simulink model "simpleTest"  (R2014a)
settings: Solver=ode45  StartTime=0.0  StopTime=10.0  RelTol=1e-3
values from neighbouring files (symbols this model uses):
  A = [0 3 4 ... (first row only)    [BJDF.m]
  B = [1;1;1]    [BJDF.m]
  C = [0 1 0;0 0 1]    [BJDF.m]
  D = [9 18;7 6;2 9]    [BJDF.m]
  f = 10    [BJDF.m]
  f1 = [-3 1 0]'    [BJDF.m]
  f2 = [1 -1/2 1/2]'    [BJDF.m]
  k = place(A,B,[-10,-11,-12])    [BJDF.m]
  pCV = CV*inv(CV'*CV)*CV'    [BJDF.m]
undefined symbols (not defined in the file or in its folder): magnitude
settings Model: Creator=sqn4594  LastModifiedBy=sqn4594

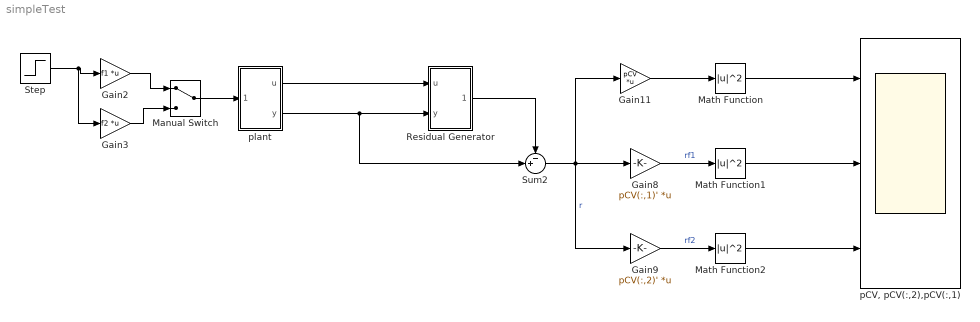
== system simpleTest ==
  Gain11 : Gain  Gain=pCV  Multiplication=Matrix(K*u)
  Gain2 : Gain  Gain=f1  Multiplication=Matrix(K*u)
  Gain3 : Gain  Gain=f2  Multiplication=Matrix(K*u)
  Gain8 : Gain  Gain=pCV(:,1)'  Multiplication=Matrix(K*u)
  Gain9 : Gain  Gain=pCV(:,2)'  Multiplication=Matrix(K*u)
  Manual Switch : ManualSwitch
  Math Function : Math  Operator=magnitude^2  SaturateOnIntegerOverflow=on
  Math Function1 : Math  Operator=magnitude^2  SaturateOnIntegerOverflow=on
  Math Function2 : Math  Operator=magnitude^2  SaturateOnIntegerOverflow=on
  Residual Generator : Subsystem
  Step : Step  Time=2  After=f  SampleTime=0
  Sum2 : Sum  Inputs=-+|
  "pCV, pCV(:,2),pCV(:,1)" : Scope  NumInputPorts=3
      settings: YMin=-5~-5~-5  YMax=5~5~5
  plant : Subsystem
  wires:
  Gain2/1 -> Manual Switch/1
  Gain3/1 -> Manual Switch/2
  Step/1 -> Gain3/1, Gain2/1
  Sum2/1 -> Gain11/1, Gain9/1, Gain8/1  "r"
  Gain8/1 -> Math Function1/1  "rf1"
  Gain9/1 -> Math Function2/1  "rf2"
  Math Function/1 -> "pCV, pCV(:,2),pCV(:,1)"/1
  Math Function1/1 -> "pCV, pCV(:,2),pCV(:,1)"/2
  Math Function2/1 -> "pCV, pCV(:,2),pCV(:,1)"/3
  Gain11/1 -> Math Function/1
  plant/2(y) -> Sum2/2, Residual Generator/2(y)
  Manual Switch/1 -> plant/1(f1/f2)
  plant/1(u) -> Residual Generator/1(u)
  Residual Generator/1(yHat) -> Sum2/1

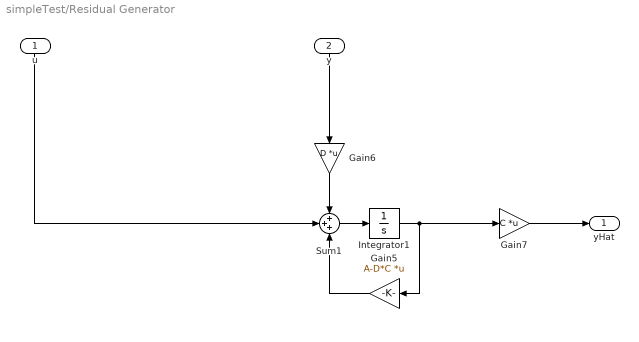
== system simpleTest/Residual Generator ==
  u : Inport
  y : Inport  Port=2
  Gain5 : Gain  Gain=A-D*C  Multiplication=Matrix(K*u)
  Gain6 : Gain  Gain=D  Multiplication=Matrix(K*u)
  Gain7 : Gain  Gain=C  Multiplication=Matrix(K*u)
  Integrator1 : Integrator
  Sum1 : Sum  Inputs=+++
  yHat : Outport
  wires:
  Gain6/1 -> Sum1/1
  Sum1/1 -> Integrator1/1
  Integrator1/1 -> Gain7/1, Gain5/1
  Gain5/1 -> Sum1/3
  Gain7/1 -> yHat/1
  u/1 -> Sum1/2
  y/1 -> Gain6/1

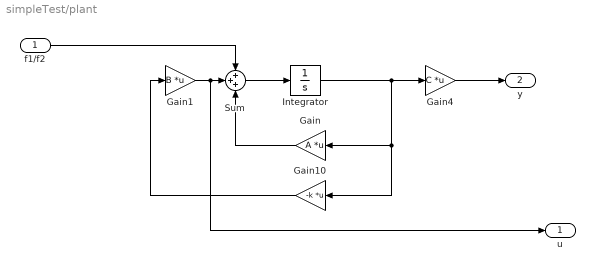
== system simpleTest/plant ==
  f1/f2 : Inport
  Gain : Gain  Gain=A  Multiplication=Matrix(K*u)
  Gain1 : Gain  Gain=B  Multiplication=Matrix(K*u)
  Gain10 : Gain  Gain=-k  Multiplication=Matrix(K*u)
  Gain4 : Gain  Gain=C  Multiplication=Matrix(K*u)
  Integrator : Integrator
  Sum : Sum  Inputs=+++
  u : Outport
  y : Outport  Port=2
  wires:
  Sum/1 -> Integrator/1
  Gain/1 -> Sum/3
  Gain1/1 -> u/1, Sum/2
  f1/f2/1 -> Sum/1
  Gain4/1 -> y/1
  Integrator/1 -> Gain4/1, Gain10/1, Gain/1
  Gain10/1 -> Gain1/1
